simulink model "Case_7bus"  (R2023b)
settings: Solver=FixedStepAuto  StartTime=0  StopTime=4  FixedStep=Ts  RelTol=1e-3
PreLoadFcn:
  | FS_Frequency=csvread('FSConfig.csv',1,0); clear FS_Result FS_Freq_point; Noise_amp=0.5e-3;load("Dome/Case_7bus/XInitial7.mat");
InitFcn:
  | FS_Frequency=csvread('FSConfig.csv',1,0); clear FS_Result FS_Freq_point; Noise_amp=0.5e-3;load("Dome/Case_7bus/XInitial7.mat");
StartFcn:
  | FS_Frequency=csvread('FSConfig.csv',1,0); clear FS_Result FS_Freq_point; Noise_amp=0.5e-3;load("Dome/Case_7bus/XInitial7.mat");
undefined symbols (not defined in the file or in its folder): ApparatusDiscreDamping, ApparatusPara, ApparatusPowerFlow, ApparatusType, OtherInputs, Ts, Wbase, x_e, Ybase, Zbase
libraries: SimplusGT x20, spsGroundLib x13, spsThreePhaseParallelRLCBranchLib x7, spsThreePhaseSeriesRLCBranchLib x7, dspindex x4, spsControlledVoltageSourceLib x3, dspsnks4 x2, simulink x1, sps_lib x1
settings Model: Creator=yz34218  LastModifiedBy=yz34218
settings DataIOCC: InitialState=XInitial7  LoadInitialState=on

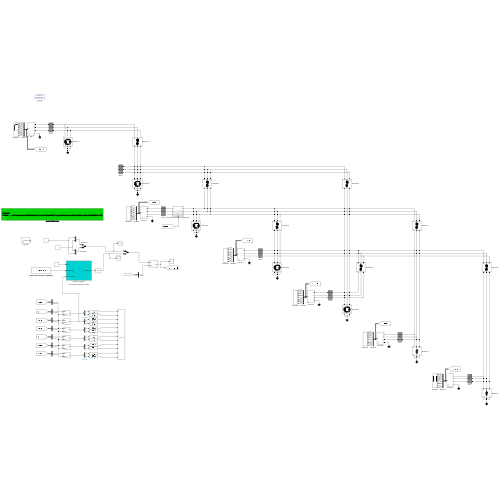
[thumbnail: Simulink's stored preview of the top-level diagram]
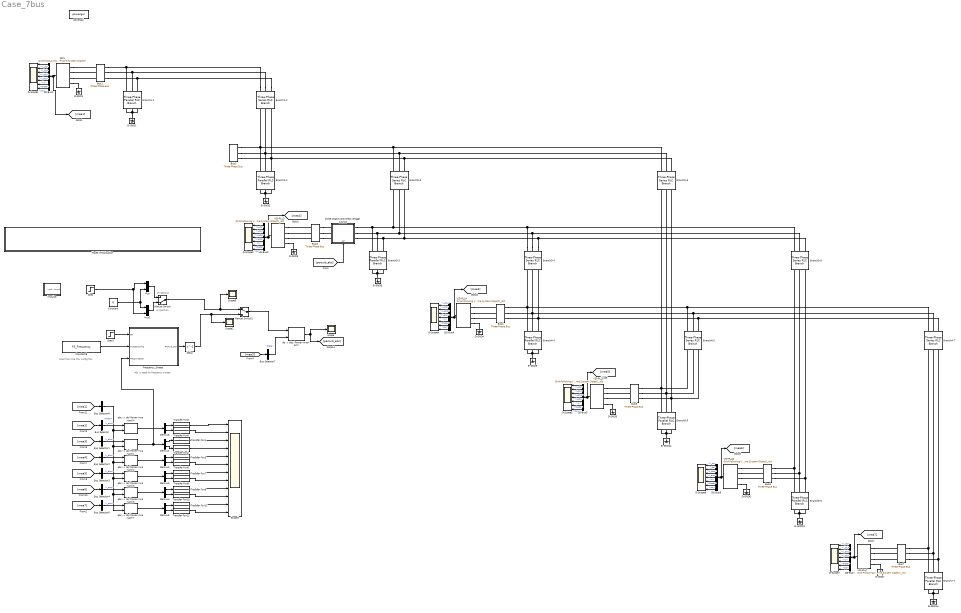
== system Case_7bus ==
  note: d-injection
  note: q-injection
  note: 40s is need for frequency sweep
  note: Input from the CSV config file.
  B-GND{1,3,6,9,12..14} (7 alike) : spsGroundLib/Ground  LConnTagsString=a
  Branch1-1 : spsThreePhaseParallelRLCBranchLib/Three-Phase Parallel RLC Branch  LConnTagsString=A|B|C  RConnTagsString=A|B|C  BranchType=RC  Resistance=(0.15273)*Zbase  Inductance=(Inf)*Zbase/Wbase  Capacitance=(0.042)*Ybase/Wbase  Measurements=None
  Branch1-2 : spsThreePhaseSeriesRLCBranchLib/Three-Phase Series RLC Branch  LConnTagsString=A|B|C  RConnTagsString=A|B|C  BranchType=RL  Resistance=(1e-06)*Zbase  Inductance=(0.039)*Zbase/Wbase  Capacitance=1e-6  Measurements=None
  Branch2-2 : spsThreePhaseParallelRLCBranchLib/Three-Phase Parallel RLC Branch  LConnTagsString=A|B|C  RConnTagsString=A|B|C  BranchType=RC  Resistance=(0.32435)*Zbase  Inductance=(Inf)*Zbase/Wbase  Capacitance=(0.042967)*Ybase/Wbase  Measurements=None
  Branch2-3 : spsThreePhaseSeriesRLCBranchLib/Three-Phase Series RLC Branch  LConnTagsString=A|B|C  RConnTagsString=A|B|C  BranchType=RL  Resistance=(0.015)*Zbase  Inductance=(0.225)*Zbase/Wbase  Capacitance=1e-6  Measurements=None
  Branch2-5 : spsThreePhaseSeriesRLCBranchLib/Three-Phase Series RLC Branch  LConnTagsString=A|B|C  RConnTagsString=A|B|C  BranchType=RL  Resistance=(0.0038)*Zbase  Inductance=(0.049)*Zbase/Wbase  Capacitance=1e-6  Measurements=None
  Branch3-3 : spsThreePhaseParallelRLCBranchLib/Three-Phase Parallel RLC Branch  LConnTagsString=A|B|C  RConnTagsString=A|B|C  BranchType=RC  Resistance=(1.4582)*Zbase  Inductance=(Inf)*Zbase/Wbase  Capacitance=(0.1491)*Ybase/Wbase  Measurements=None
  Branch3-4 : spsThreePhaseSeriesRLCBranchLib/Three-Phase Series RLC Branch  LConnTagsString=A|B|C  RConnTagsString=A|B|C  BranchType=RL  Resistance=(0.005)*Zbase  Inductance=(0.076)*Zbase/Wbase  Capacitance=1e-6  Measurements=None
  Branch3-6 : spsThreePhaseSeriesRLCBranchLib/Three-Phase Series RLC Branch  LConnTagsString=A|B|C  RConnTagsString=A|B|C  BranchType=RL  Resistance=(0.002)*Zbase  Inductance=(0.02)*Zbase/Wbase  Capacitance=1e-6  Measurements=None
  Branch4-4 : spsThreePhaseParallelRLCBranchLib/Three-Phase Parallel RLC Branch  LConnTagsString=A|B|C  RConnTagsString=A|B|C  BranchType=RC  Resistance=(1.4454)*Zbase  Inductance=(Inf)*Zbase/Wbase  Capacitance=(0.1142)*Ybase/Wbase  Measurements=None
  Branch4-5 : spsThreePhaseSeriesRLCBranchLib/Three-Phase Series RLC Branch  LConnTagsString=A|B|C  RConnTagsString=A|B|C  BranchType=RL  Resistance=(0.003)*Zbase  Inductance=(0.038)*Zbase/Wbase  Capacitance=1e-6  Measurements=None
  Branch4-7 : spsThreePhaseSeriesRLCBranchLib/Three-Phase Series RLC Branch  LConnTagsString=A|B|C  RConnTagsString=A|B|C  BranchType=RL  Resistance=(0.004)*Zbase  Inductance=(0.04)*Zbase/Wbase  Capacitance=1e-6  Measurements=None
  Branch5-5 : spsThreePhaseParallelRLCBranchLib/Three-Phase Parallel RLC Branch  LConnTagsString=A|B|C  RConnTagsString=A|B|C  BranchType=RC  Resistance=(2.3723)*Zbase  Inductance=(Inf)*Zbase/Wbase  Capacitance=(0.1792)*Ybase/Wbase  Measurements=None
  Branch6-6 : spsThreePhaseParallelRLCBranchLib/Three-Phase Parallel RLC Branch  LConnTagsString=A|B|C  RConnTagsString=A|B|C  BranchType=C  Resistance=(Inf)*Zbase  Inductance=(Inf)*Zbase/Wbase  Capacitance=(0.2)*Ybase/Wbase  Measurements=None
  Branch7-7 : spsThreePhaseParallelRLCBranchLib/Three-Phase Parallel RLC Branch  LConnTagsString=A|B|C  RConnTagsString=A|B|C  BranchType=C  Resistance=(Inf)*Zbase  Inductance=(Inf)*Zbase/Wbase  Capacitance=(0.2)*Ybase/Wbase  Measurements=None
  Bus Selector{,1..5} (6 alike) : BusSelector  OutputSignals=i_abc
  Bus Selector6 : BusSelector  OutputSignals=theta
  Bus Selector7 : BusSelector  OutputSignals=theta
  Bus{1..7} (7 alike) : SimplusGT/Three-Phase Bus  Vbase=1  Sbase=1
      settings: SourceProductName=Simplus Grid Tool
  Constant : Constant  Value=0
  Constant8 : Constant  Value=FS_Frequency
  D-GND{1,3..7} (6 alike) : spsGroundLib/Ground  LConnTagsString=a
  D-Scope{1,3..7} (6 alike) : Scope  NumInputPorts=7
  DS-Bus{1,3..7} (6 alike) : BusSelector  OutputSignals=v_dq,i_dq,v_abc,i_abc,w,theta,pq
  Delay : Delay  DelayLength=1
  Demux{1..5,8} (6 alike) : Demux  Outputs=2
  Frequency_Sweep : Subsystem  mask{Gain=0.01, Interval=0}
      mask prompts: Gain "Output Gain"; Interval "Injection Interval"
  Manual Switch : ManualSwitch  CurrentSetting=0
  Manual Switch1 : ManualSwitch
  Model Initialization : Subsystem  mask(Model Functions){InitFcnVar=FS_Frequency=csvread('FSConfig.csv',1,0); clear FS_Result FS_Freq_point; Noise_amp=0.5e-3;load("Dome/Case_7bus/XInitial7.mat");}
      mask prompts: InitFcnVar "InitFcn"
      mask init:
      | set_param(bdroot, 'PreLoadFcn', InitFcnVar);
      | set_param(bdroot, 'InitFcn', InitFcnVar);
      | set_param(bdroot, 'StartFcn', InitFcnVar);
      | PLF = get_param(bdroot, 'PreLoadFcn');
      | IF = get_param(bdroot, 'InitFcn');
      | SF = get_param(bdroot, 'StartFcn');
      | 
      | 
      | pos = get_param(gcb, 'Position');
      | width = pos(3) - pos(1); height = pos(4) - pos(2);
      mask Display:
      | text(5, height*0.5, [ ...
      | upper(bdroot) '\n' ...
      | '- InitFcn. . . . . '  get_param(bdroot, 'InitFcn')  ...
      | ], ...
      | 'horizontalAlignment', 'left', 'verticalAlignment', 'middle') ;
  Mux : Mux  Inputs=2
  Mux1 : Mux  Inputs=2
  SM1 : SimplusGT/Synchronous Machine (dq-Frame System Object)  Ts=Ts  Sbase=Sbase  Vbase=Vbase  Wbase=Wbase  ApparatusType=ApparatusType{1}  ApparatusPara=ApparatusPara{1}  PowerFlow=ApparatusPowerFlow{1}  x0=x_e{1}  OtherInputs=OtherInputs{1}  DiscreMethod=Hybrid Trapezoidal  EnableInsideModification=off  DiscreDampingFlag=on  DiscreDampingValue=ApparatusDiscreDamping{1}  LinearizationTimes=1  DirectFeedthrough=off
      settings: SourceProductName=Simplus Grid Tool
  Scope : Scope
  Scope2 : Scope
  Scope3 : Scope  NumInputPorts=12
  Scope5 : Scope
  Step : Step  After=2e-2  SampleTime=0
  Step1 : Step  Time=2  SampleTime=0
  Transfer Fcn{1..12} (12 alike) : TransferFcn  Denominator=[1/(2*pi*200) 1]
  VSI-PLL3 : SimplusGT/Grid-Following Voltage-Source Inverter (dq-Frame System Object)_old  Ts=Ts  Sbase=Sbase  Vbase=Vbase  Wbase=Wbase  ApparatusType=ApparatusType{3}  ApparatusPara=ApparatusPara{3}  PowerFlow=ApparatusPowerFlow{3}  x0=x_e{3}  OtherInputs=OtherInputs{3}  DiscreMethod=Hybrid Trapezoidal  EnableInsideModification=off  DiscreDampingFlag=on  DiscreDampingValue=ApparatusDiscreDamping{3}  LinearizationTimes=1  DirectFeedthrough=off
      settings: SourceProductName=Simplus Grid Tool
  VSI-PLL4 : SimplusGT/Grid-Following Voltage-Source Inverter (dq-Frame System Object)_old  Ts=Ts  Sbase=Sbase  Vbase=Vbase  Wbase=Wbase  ApparatusType=ApparatusType{4}  ApparatusPara=ApparatusPara{4}  PowerFlow=ApparatusPowerFlow{4}  x0=x_e{4}  OtherInputs=OtherInputs{4}  DiscreMethod=Hybrid Trapezoidal  EnableInsideModification=off  DiscreDampingFlag=on  DiscreDampingValue=ApparatusDiscreDamping{4}  LinearizationTimes=1  DirectFeedthrough=off
      settings: SourceProductName=Simplus Grid Tool
  VSI-PLL5 : SimplusGT/Grid-Following Voltage-Source Inverter (dq-Frame System Object)_old  Ts=Ts  Sbase=Sbase  Vbase=Vbase  Wbase=Wbase  ApparatusType=ApparatusType{5}  ApparatusPara=ApparatusPara{5}  PowerFlow=ApparatusPowerFlow{5}  x0=x_e{5}  OtherInputs=OtherInputs{5}  DiscreMethod=Hybrid Trapezoidal  EnableInsideModification=off  DiscreDampingFlag=on  DiscreDampingValue=ApparatusDiscreDamping{5}  LinearizationTimes=1  DirectFeedthrough=off
      settings: SourceProductName=Simplus Grid Tool
  VSI-PLL6 : SimplusGT/Grid-Following Voltage-Source Inverter (dq-Frame System Object)_old  Ts=Ts  Sbase=Sbase  Vbase=Vbase  Wbase=Wbase  ApparatusType=ApparatusType{6}  ApparatusPara=ApparatusPara{6}  PowerFlow=ApparatusPowerFlow{6}  x0=x_e{6}  OtherInputs=OtherInputs{6}  DiscreMethod=Hybrid Trapezoidal  EnableInsideModification=off  DiscreDampingFlag=on  DiscreDampingValue=ApparatusDiscreDamping{6}  LinearizationTimes=1  DirectFeedthrough=off
      settings: SourceProductName=Simplus Grid Tool
  VSI-PLL7 : SimplusGT/Grid-Following Voltage-Source Inverter (dq-Frame System Object)_old  Ts=Ts  Sbase=Sbase  Vbase=Vbase  Wbase=Wbase  ApparatusType=ApparatusType{7}  ApparatusPara=ApparatusPara{7}  PowerFlow=ApparatusPowerFlow{7}  x0=x_e{7}  OtherInputs=OtherInputs{7}  DiscreMethod=Hybrid Trapezoidal  EnableInsideModification=off  DiscreDampingFlag=on  DiscreDampingValue=ApparatusDiscreDamping{7}  LinearizationTimes=1  DirectFeedthrough=off
      settings: SourceProductName=Simplus Grid Tool
  abc -> dq (Power-Invariant){1..4,6..7} (6 alike) : SimplusGT/abc -> dq (Power-Invariant)  SystemSampleTime=-1  VariantActivationTime=update diagram  AllowFlexibleInterface=on  Latency=0  AutoFrameSizeCalculation=off
      settings: SourceProductName=Simplus Grid Tool
  "dq -> abc (Power-Invariant)" : SimplusGT/dq -> abc (Power-Invariant)  SystemSampleTime=-1  VariantActivationTime=update diagram  AllowFlexibleInterface=on  Latency=0  AutoFrameSizeCalculation=off
      settings: SourceProductName=Simplus Grid Tool
  impulse : Subsystem  mask{Amp=2e-2, Tstart=1, Ti=1e-3}
      mask prompts: Amp "amplitude"; Ti "Tinterval"
  powergui : sps_lib/powergui  Priority=1  SimulationMode=Discrete  SampleTime=Ts  frequency=60  Iterations=50  frequencyindice=0  Pbase=100e6  ErrMax=1e-4  UnitsV=kV  UnitsW=MW  buscounter=0  FunctionMessages=off  echomessages=off  EnableUseOfTLC=off  CurrentSourceSwitches=off  DisableSnubberDevices=off  DisableRonSwitches=off  DisableVfSwitches=off  DisplayEquations=off  AutomaticDiscreteSolvers=off  SolverType=Tustin/Backward Euler (TBE)  Interpol=off  ExternalGateDelay=off  methode=off  Ts=100  x0status=blocks  SPID=on  SwTol=0  HookPort=off  NonlinearTolerance=1e-4  nMaxIteration=100  ContinueOnMaxIteration=off  RestoreLinks=warning  ResistiveCurrentMeasurement=off  Frange=[0:2:500]  Ylog=off  Xlog=on  ShowGrid=off  save=off  variable=ZData  structure=0  ZoomFFT=off  StartTime=0.0  cycles=1  DisplayStyle=1  fundamental=60  FreqAxis=off  MaxFrequency=1000  frequencyindicesteady=1  RmsSteady=1  display=off
  three-phase controlled voltage source : Subsystem
      settings: PortSchema="{\"entries\":[{\"content\":{\"sides\":[{\"content\":{\"connectorIds\":[\"LConn1\",\"LConn2\",\"LConn3\"]},\"type\":\"ConnectorPlacement.EquallySpacedRectSide\",\"uuid\":\"6f603e87-6b2e-4585-ad3a-55936445c397\"},{\"content\":{\"connectorIds\":[\"RConn1\",\"RConn2\",\"RConn3\"],\"side\":\"RIGHT\"},\"type\":\"ConnectorPlacement.EquallySpacedRectSide\",\"uuid\":\"08c5aebc-ed45-455a-9198-e657d358a757\"},{\"content\":{\"side\":\"TOP\"},\"type\":\"ConnectorPlacement.EquallySpacedRectSide\",\"uuid\":\"90e892ab-d7d1-4f2e-b125-0b742fd1657c\"},{\"content\":{\"connectorIds\":[\"In1\"],\"side\":\"BOTTOM\"},\"type\":\"ConnectorPlacement.EquallySpacedRectSide\",\"uuid\":\"ba12d237-2ee0-4e5a-b3d4-1de3f90cbef1\"}]},\"type\":\"ConnectorPlacement.EquallySpacedConnector\",\"uuid\":\"0150c08c-ed05-4e99-aa85-f9e708dbbe93\"}],\"packageUris\":[\"http://schema.mathworks.com/mf0/Connector/R2020b\"],\"version\":\"1.0\"}"
  wires:
  SM1/1 -> [mea1], DS-Bus1/1
  DS-Bus1/1 -> D-Scope1/1  "<v_dq>"
  DS-Bus1/2 -> D-Scope1/2  "<i_dq>"
  DS-Bus1/3 -> D-Scope1/3  "<v_abc>"
  DS-Bus1/4 -> D-Scope1/4  "<i_abc>"
  DS-Bus1/5 -> D-Scope1/5  "<w>"
  DS-Bus1/6 -> D-Scope1/6  "<theta>"
  DS-Bus1/7 -> D-Scope1/7  "<pq>"
  VSI-PLL3/1 -> [mea3], DS-Bus3/1
  DS-Bus3/1 -> D-Scope3/1  "<v_dq>"
  DS-Bus3/2 -> D-Scope3/2  "<i_dq>"
  DS-Bus3/3 -> D-Scope3/3  "<v_abc>"
  DS-Bus3/4 -> D-Scope3/4  "<i_abc>"
  DS-Bus3/5 -> D-Scope3/5  "<w>"
  DS-Bus3/6 -> D-Scope3/6  "<theta>"
  DS-Bus3/7 -> D-Scope3/7  "<pq>"
  VSI-PLL4/1 -> [mea4], DS-Bus4/1
  DS-Bus4/1 -> D-Scope4/1  "<v_dq>"
  DS-Bus4/2 -> D-Scope4/2  "<i_dq>"
  DS-Bus4/3 -> D-Scope4/3  "<v_abc>"
  DS-Bus4/4 -> D-Scope4/4  "<i_abc>"
  DS-Bus4/5 -> D-Scope4/5  "<w>"
  DS-Bus4/6 -> D-Scope4/6  "<theta>"
  DS-Bus4/7 -> D-Scope4/7  "<pq>"
  VSI-PLL5/1 -> [mea5], DS-Bus5/1
  DS-Bus5/1 -> D-Scope5/1  "<v_dq>"
  DS-Bus5/2 -> D-Scope5/2  "<i_dq>"
  DS-Bus5/3 -> D-Scope5/3  "<v_abc>"
  DS-Bus5/4 -> D-Scope5/4  "<i_abc>"
  DS-Bus5/5 -> D-Scope5/5  "<w>"
  DS-Bus5/6 -> D-Scope5/6  "<theta>"
  DS-Bus5/7 -> D-Scope5/7  "<pq>"
  VSI-PLL6/1 -> [mea6], DS-Bus6/1
  DS-Bus6/1 -> D-Scope6/1  "<v_dq>"
  DS-Bus6/2 -> D-Scope6/2  "<i_dq>"
  DS-Bus6/3 -> D-Scope6/3  "<v_abc>"
  DS-Bus6/4 -> D-Scope6/4  "<i_abc>"
  DS-Bus6/5 -> D-Scope6/5  "<w>"
  DS-Bus6/6 -> D-Scope6/6  "<theta>"
  DS-Bus6/7 -> D-Scope6/7  "<pq>"
  VSI-PLL7/1 -> [mea7], DS-Bus7/1
  DS-Bus7/1 -> D-Scope7/1  "<v_dq>"
  DS-Bus7/2 -> D-Scope7/2  "<i_dq>"
  DS-Bus7/3 -> D-Scope7/3  "<v_abc>"
  DS-Bus7/4 -> D-Scope7/4  "<i_abc>"
  DS-Bus7/5 -> D-Scope7/5  "<w>"
  DS-Bus7/6 -> D-Scope7/6  "<theta>"
  DS-Bus7/7 -> D-Scope7/7  "<pq>"
  [perturb_abc] -> three-phase controlled voltage source/1(ref)
  Frequency_Sweep/1(Perturb_DQ) -> Delay/1
  Manual Switch/1 -> Scope5/1, Manual Switch1/1
  Constant8/1 -> Frequency_Sweep/2(SweepConfig)
  Mux/1 -> Manual Switch/1
  Step/1 -> Mux1/2, Mux/1
  Delay/1 -> Scope2/1, Manual Switch1/2
  Step1/1 -> Frequency_Sweep/1(EN)
  Manual Switch1/1 -> "dq -> abc (Power-Invariant)"/1
  "dq -> abc (Power-Invariant)"/1 -> Scope/1, [perturb_abc]
  Constant/1 -> Mux/2, Mux1/1
  "abc -> dq (Power-Invariant)1"/1 -> Frequency_Sweep/3(ResponseDQ), Demux1/1
  Mux1/1 -> Manual Switch/2
  [mea1] -> Bus Selector/1
  [mea3] -> Bus Selector1/1
  [mea4] -> Bus Selector2/1
  [mea5] -> Bus Selector3/1
  [mea6] -> Bus Selector4/1
  [mea7] -> Bus Selector5/1
  [mea1] -> Bus Selector6/1
  Bus Selector/1 -> "abc -> dq (Power-Invariant)4"/1  "<i_abc>"
  Bus Selector1/1 -> "abc -> dq (Power-Invariant)1"/1  "<i_abc>"
  Bus Selector2/1 -> "abc -> dq (Power-Invariant)2"/1  "<i_abc>"
  Bus Selector3/1 -> "abc -> dq (Power-Invariant)3"/1  "<i_abc>"
  Bus Selector4/1 -> "abc -> dq (Power-Invariant)6"/1  "<i_abc>"
  Bus Selector5/1 -> "abc -> dq (Power-Invariant)7"/1  "<i_abc>"
  Bus Selector6/1 -> "abc -> dq (Power-Invariant)7"/2, "abc -> dq (Power-Invariant)6"/2, "abc -> dq (Power-Invariant)3"/2, "abc -> dq (Power-Invariant)2"/2, "abc -> dq (Power-Invariant)1"/2, "abc -> dq (Power-Invariant)4"/2  "<theta>"
  "abc -> dq (Power-Invariant)4"/1 -> Demux8/1
  "abc -> dq (Power-Invariant)2"/1 -> Demux2/1
  "abc -> dq (Power-Invariant)3"/1 -> Demux3/1
  "abc -> dq (Power-Invariant)6"/1 -> Demux4/1
  "abc -> dq (Power-Invariant)7"/1 -> Demux5/1
  Demux8/1 -> Transfer Fcn3/1
  Demux8/2 -> Transfer Fcn4/1
  Demux2/1 -> Transfer Fcn5/1
  Demux2/2 -> Transfer Fcn6/1
  Demux3/1 -> Transfer Fcn7/1
  Demux3/2 -> Transfer Fcn8/1
  Demux4/1 -> Transfer Fcn9/1
  Demux4/2 -> Transfer Fcn10/1
  Demux5/1 -> Transfer Fcn11/1
  Demux5/2 -> Transfer Fcn12/1
  [mea3] -> Bus Selector7/1
  Bus Selector7/1 -> "dq -> abc (Power-Invariant)"/2  "<theta>"
  Demux1/1 -> Transfer Fcn1/1
  Transfer Fcn1/1 -> Scope3/3
  Demux1/2 -> Transfer Fcn2/1
  Transfer Fcn2/1 -> Scope3/4
  Transfer Fcn3/1 -> Scope3/1
  Transfer Fcn4/1 -> Scope3/2
  Transfer Fcn5/1 -> Scope3/5
  Transfer Fcn6/1 -> Scope3/6
  Transfer Fcn7/1 -> Scope3/7
  Transfer Fcn8/1 -> Scope3/8
  Transfer Fcn9/1 -> Scope3/9
  Transfer Fcn10/1 -> Scope3/10
  Transfer Fcn11/1 -> Scope3/11
  Transfer Fcn12/1 -> Scope3/12
  connections:
  SM1/LConn4 -- D-GND1/LConn1
  VSI-PLL3/LConn4 -- D-GND3/LConn1
  VSI-PLL4/LConn4 -- D-GND4/LConn1
  VSI-PLL5/LConn4 -- D-GND5/LConn1
  VSI-PLL6/LConn4 -- D-GND6/LConn1
  VSI-PLL7/LConn4 -- D-GND7/LConn1
  Branch1-1/RConn1 -- Branch1-1/RConn2 -- Branch1-1/RConn3 -- B-GND1/LConn1
  Branch2-2/RConn1 -- Branch2-2/RConn2 -- Branch2-2/RConn3 -- B-GND3/LConn1
  Branch3-3/RConn1 -- Branch3-3/RConn2 -- Branch3-3/RConn3 -- B-GND6/LConn1
  Branch4-4/RConn1 -- Branch4-4/RConn2 -- Branch4-4/RConn3 -- B-GND9/LConn1
  Branch5-5/RConn1 -- Branch5-5/RConn2 -- Branch5-5/RConn3 -- B-GND12/LConn1
  Branch6-6/RConn1 -- Branch6-6/RConn2 -- Branch6-6/RConn3 -- B-GND13/LConn1
  Branch7-7/RConn1 -- Branch7-7/RConn2 -- Branch7-7/RConn3 -- B-GND14/LConn1
  Branch1-2/RConn1 -- Bus2/RConn1 -- Branch2-2/LConn1 -- Branch2-5/LConn1 -- Branch2-3/LConn1
  Branch1-2/RConn2 -- Bus2/RConn2 -- Branch2-2/LConn2 -- Branch2-5/LConn2 -- Branch2-3/LConn2
  Branch1-2/RConn3 -- Bus2/RConn3 -- Branch2-2/LConn3 -- Branch2-5/LConn3 -- Branch2-3/LConn3
  Branch1-2/LConn1 -- Bus1/RConn1 -- Branch1-1/LConn1
  Branch1-2/LConn2 -- Bus1/RConn2 -- Branch1-1/LConn2
  Branch1-2/LConn3 -- Bus1/RConn3 -- Branch1-1/LConn3
  Branch3-4/LConn1 -- three-phase controlled voltage source/RConn1 -- Branch3-3/LConn1 -- Branch2-3/RConn1 -- Branch3-6/LConn1
  Branch3-4/LConn2 -- three-phase controlled voltage source/RConn2 -- Branch3-3/LConn2 -- Branch2-3/RConn2 -- Branch3-6/LConn2
  Branch3-4/LConn3 -- three-phase controlled voltage source/RConn3 -- Branch3-3/LConn3 -- Branch2-3/RConn3 -- Branch3-6/LConn3
  Branch2-5/RConn1 -- Bus5/RConn1 -- Branch5-5/LConn1 -- Branch4-5/RConn1
  Branch2-5/RConn2 -- Bus5/RConn2 -- Branch5-5/LConn2 -- Branch4-5/RConn2
  Branch2-5/RConn3 -- Bus5/RConn3 -- Branch5-5/LConn3 -- Branch4-5/RConn3
  Branch3-4/RConn1 -- Bus4/RConn1 -- Branch4-4/LConn1 -- Branch4-7/LConn1 -- Branch4-5/LConn1
  Branch3-4/RConn2 -- Bus4/RConn2 -- Branch4-4/LConn2 -- Branch4-7/LConn2 -- Branch4-5/LConn2
  Branch3-4/RConn3 -- Bus4/RConn3 -- Branch4-4/LConn3 -- Branch4-7/LConn3 -- Branch4-5/LConn3
  Branch3-6/RConn1 -- Bus6/RConn1 -- Branch6-6/LConn1
  Branch3-6/RConn2 -- Bus6/RConn2 -- Branch6-6/LConn2
  Branch3-6/RConn3 -- Bus6/RConn3 -- Branch6-6/LConn3
  Branch4-7/RConn1 -- Bus7/RConn1 -- Branch7-7/LConn1
  Branch4-7/RConn2 -- Bus7/RConn2 -- Branch7-7/LConn2
  Branch4-7/RConn3 -- Bus7/RConn3 -- Branch7-7/LConn3
  SM1/LConn1 -- Bus1/LConn1
  SM1/LConn2 -- Bus1/LConn2
  SM1/LConn3 -- Bus1/LConn3
  VSI-PLL3/LConn1 -- Bus3/LConn1
  VSI-PLL3/LConn2 -- Bus3/LConn2
  VSI-PLL3/LConn3 -- Bus3/LConn3
  VSI-PLL4/LConn1 -- Bus4/LConn1
  VSI-PLL4/LConn2 -- Bus4/LConn2
  VSI-PLL4/LConn3 -- Bus4/LConn3
  VSI-PLL5/LConn1 -- Bus5/LConn1
  VSI-PLL5/LConn2 -- Bus5/LConn2
  VSI-PLL5/LConn3 -- Bus5/LConn3
  VSI-PLL6/LConn1 -- Bus6/LConn1
  VSI-PLL6/LConn2 -- Bus6/LConn2
  VSI-PLL6/LConn3 -- Bus6/LConn3
  VSI-PLL7/LConn1 -- Bus7/LConn1
  VSI-PLL7/LConn2 -- Bus7/LConn2
  VSI-PLL7/LConn3 -- Bus7/LConn3
  Bus3/RConn1 -- three-phase controlled voltage source/LConn1
  Bus3/RConn2 -- three-phase controlled voltage source/LConn2
  Bus3/RConn3 -- three-phase controlled voltage source/LConn3

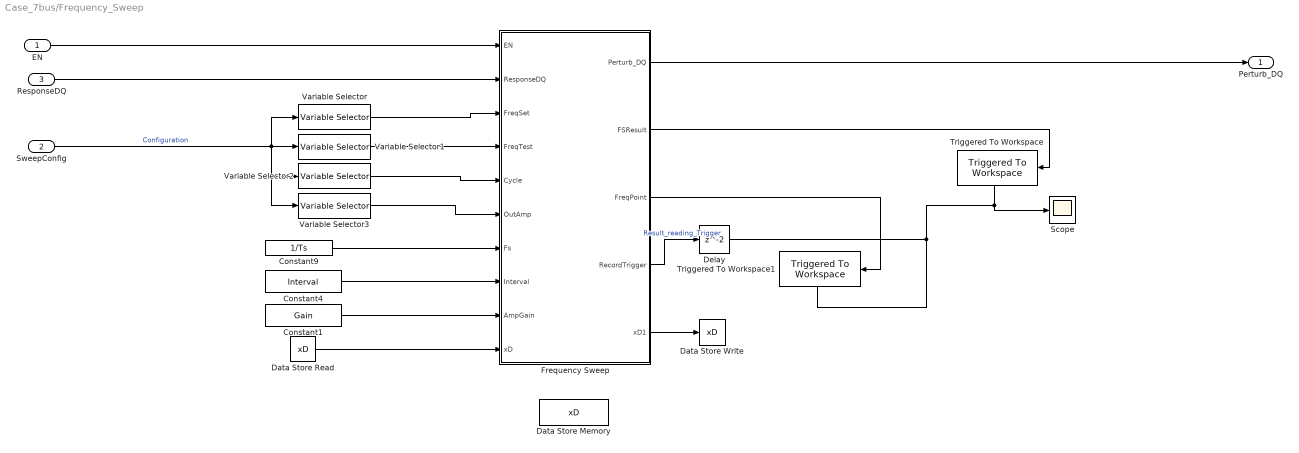
== system Case_7bus/Frequency_Sweep ==
  EN : Inport
  SweepConfig : Inport  Port=2
  ResponseDQ : Inport  Port=3
  Constant1 : Constant  Value=Gain
  Constant4 : Constant  Value=Interval
  Constant9 : Constant  Value=1/Ts
  Data Store Memory : DataStoreMemory  DataStoreName=xD  WriteAfterWriteMsg=warning  InitialValue=zeros(1,16)  ShowAdditionalParam=off
  Data Store Read : DataStoreRead  DataStoreName=xD  IndexOptions=Index vector (dialog)  Indices=1  OutputSizes=1
  Data Store Write : DataStoreWrite  DataStoreName=xD  IndexOptions=Index vector (dialog)  Indices=1  OutputSizes=1
  Delay : Delay
  Frequency Sweep : MATLAB Function  TreatAsAtomicUnit=on
  Scope : Scope
  Triggered To Workspace : dspsnks4/Triggered To Workspace  TriggerType=Rising edge  VariableName=FS_Result  Buffer=5000  Save2DMode=2-D array (concatenate along first dimension)
      settings: FixptAsFi=off
  Triggered To Workspace1 : dspsnks4/Triggered To Workspace  TriggerType=Rising edge  VariableName=FS_Freq_point  Buffer=5000  Save2DMode=2-D array (concatenate along first dimension)
      settings: FixptAsFi=off
  Variable Selector : dspindex/Variable Selector  NumInputs=1  rowsOrCols=Columns  IdxMode=Fixed  Elements=1  ZerOneIdxMode=One-based  errmode=Clip Index  FillMode=on  FillValues=0
  Variable Selector1 : dspindex/Variable Selector  NumInputs=1  rowsOrCols=Columns  IdxMode=Fixed  Elements=2  ZerOneIdxMode=One-based  errmode=Clip Index  FillMode=on  FillValues=0
  Variable Selector2 : dspindex/Variable Selector  NumInputs=1  rowsOrCols=Columns  IdxMode=Fixed  Elements=3  ZerOneIdxMode=One-based  errmode=Clip Index  FillMode=on  FillValues=0
  Variable Selector3 : dspindex/Variable Selector  NumInputs=1  rowsOrCols=Columns  IdxMode=Fixed  Elements=4  ZerOneIdxMode=One-based  errmode=Clip Index  FillMode=on  FillValues=0
  Perturb_DQ : Outport
  wires:
  Variable Selector2/1 -> Frequency Sweep/5(Cycle)
  Frequency Sweep/2(FSResult) -> Triggered To Workspace/1
  Frequency Sweep/4(RecordTrigger) -> Delay/1  "Result_reading_Trigger"
  Constant4/1 -> Frequency Sweep/8(Interval)
  Frequency Sweep/5(xD1) -> Data Store Write/1
  Variable Selector3/1 -> Frequency Sweep/6(OutAmp)
  Variable Selector1/1 -> Frequency Sweep/4(FreqTest)
  SweepConfig/1 -> Variable Selector3/1, Variable Selector2/1, Variable Selector1/1, Variable Selector/1  "Configuration"
  ResponseDQ/1 -> Frequency Sweep/2(ResponseDQ)
  Variable Selector/1 -> Frequency Sweep/3(FreqSet)
  Frequency Sweep/3(FreqPoint) -> Triggered To Workspace1/1
  Data Store Read/1 -> Frequency Sweep/10(xD)
  Constant9/1 -> Frequency Sweep/7(Fs)
  Frequency Sweep/1(Perturb_DQ) -> Perturb_DQ/1
  EN/1 -> Frequency Sweep/1(EN)
  Delay/1 -> Triggered To Workspace/Trigger, Scope/1, Triggered To Workspace1/Trigger
  Constant1/1 -> Frequency Sweep/9(AmpGain)

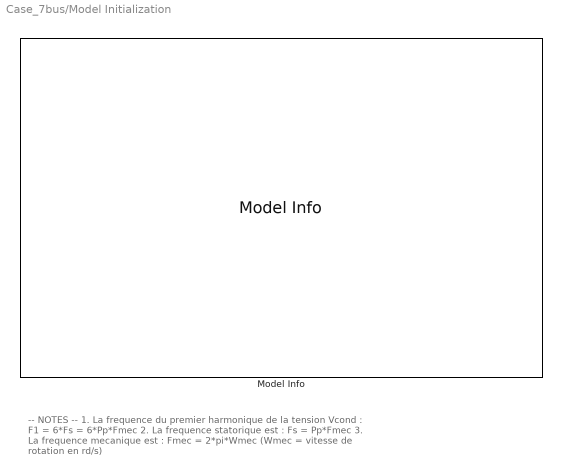
== system Case_7bus/Model Initialization ==
  note: -- NOTES --
      | 1. La frequence du premier harmonique de la tension Vcond :
      |     F1 = 6*Fs = 6*Pp*Fmec
      | 2. La frequence statorique est :
      |     Fs = Pp*Fmec
      | 3. La frequence mecanique est :
      |     Fmec = 2*pi*Wmec  (Wmec = vitesse de rotation en rd/s)
  Model Info : simulink/Model-Wide Utilities/Model Info  Frame=on  DisplayStringWithTags=|  HorizontalTextAlignment=Left  LeftAlignmentValue=0.02
      | - Version <<< %<ModelVersion> >>>
      | 
      | - Description :
      | %<Description>
      | 
      | - Created by :     %<Creator>
      | - Creation date : %<Created>
      | - Modified by :    %<ModifiedBy>
      | - Last modif. :     %<LastModificationDate>

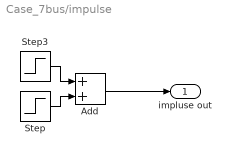
== system Case_7bus/impulse ==
  Add : Sum
  Step : Step  Time=Tstart+Ti  After=-Amp  SampleTime=0
  Step3 : Step  Time=Tstart  After=Amp  SampleTime=0
  impluse out : Outport
  wires:
  Step/1 -> Add/2
  Step3/1 -> Add/1
  Add/1 -> impluse out/1

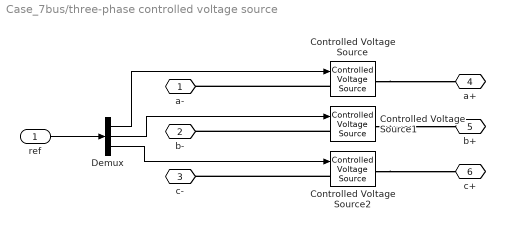
== system Case_7bus/three-phase controlled voltage source ==
  ref : Inport
  Controlled Voltage Source : spsControlledVoltageSourceLib/Controlled Voltage Source  Initialize=on  Source_Type=AC  Amplitude=0  Phase=0  Frequency=0  Measurements=None
  Controlled Voltage Source1 : spsControlledVoltageSourceLib/Controlled Voltage Source  Initialize=on  Source_Type=AC  Amplitude=0  Phase=0  Frequency=0  Measurements=None
  Controlled Voltage Source2 : spsControlledVoltageSourceLib/Controlled Voltage Source  Initialize=on  Source_Type=AC  Amplitude=0  Phase=0  Frequency=0  Measurements=None
  Demux : Demux  Outputs=3
  a- : PMIOPort  Side=Left
  b- : PMIOPort  Port=2  Side=Left
  c- : PMIOPort  Port=3  Side=Left
  a+ : PMIOPort  Port=4  Side=Right
  b+ : PMIOPort  Port=5  Side=Right
  c+ : PMIOPort  Port=6  Side=Right
  wires:
  Demux/2 -> Controlled Voltage Source1/1
  Demux/3 -> Controlled Voltage Source2/1
  ref/1 -> Demux/1
  Demux/1 -> Controlled Voltage Source/1
  connections:
  Controlled Voltage Source/LConn1 -- a-/RConn1
  Controlled Voltage Source1/RConn1 -- b+/RConn1
  Controlled Voltage Source1/LConn1 -- b-/RConn1
  Controlled Voltage Source/RConn1 -- a+/RConn1
  Controlled Voltage Source2/RConn1 -- c+/RConn1
  Controlled Voltage Source2/LConn1 -- c-/RConn1

== matlab function Case_7bus/Frequency_Sweep/Frequency Sweep ==
  data: EN input; Perturb_DQ output; ResponseDQ input size=[1 2]; FreqSet input; FreqTest input; Cycle input; OutAmp input; Fs input; Interval input; AmpGain input; xD input; FSResult output; FreqPoint output; RecordTrigger output; xD1 output
function [Perturb_DQ, FSResult, FreqPoint, RecordTrigger, xD1] = fcn(EN,ResponseDQ, FreqSet, FreqTest, Cycle, OutAmp, Fs, Interval, AmpGain, xD)
% State variables:
% xD0: case;        xD1:N; total sample points for one period
% xD2:-N;           xD3:n ,sample point count      xD4:k, for cycle count
% xD5: Out_Re       xD6:Out_Im;
% xD7: Sum_Re_d      xD8:Sum_Im_d     xD9:Sum_Re_q     xD10:Sum_Im_q
% xD11, xD12, xD13, xD14----xD7,xD8,xD9,xD10 * dt
% xD15: t, for waiting

% read states
CaseK=xD(1); % case
Ns=xD(2); % total time steps for the set frequency
Nt=xD(3); % total time steps for the tested (calculated) frequency
n=xD(4); % sample point count
kc=xD(5);   % CycleCount
OutD=xD(6); %   Output
OutQ=xD(7);
SumDRe=xD(8); % Integration
SumDIm=xD(9);
SumQRe=xD(10);
SumQIm=xD(11);
FinalDRe=xD(12); % Final Result (complex number)
FinalDIm=xD(13);
FinalQRe=xD(14);
FinalQIm=xD(15);
TWait=xD(16); % wait time

FrequencyNum=length(FreqSet);

if AmpGain==0
    error('gain must not be zero');
end

%% Main Loop
if EN==0   % if Enable 0, reset all variables
    OutD=0;
    OutQ=0;
else
    switch CaseK
        case 0 % the very first round
            kc=1;
            CaseK=1;
        case 1
            if kc>FrequencyNum         %sweep finished. Go to case 9
                OutD=0;
                OutQ=0;   
                CaseK=9; 
            elseif Cycle(kc)==0  % if this frequency is skipped
                kc=kc+1;
            else   
                % prepare to sweep D axis this frequency
                SumDRe=0;
                SumDIm=0;
                SumQRe=0;
                SumQIm=0;
                TWait=0;
                n=0;
                % total time steps for this frequency
                Ns = Fs/FreqSet(kc)*Cycle(kc); % for output count
                Nt = Fs/FreqTest(kc)*Cycle(kc); % for frequency test count
                OutD=OutAmp(kc)*sin(2*pi*Cycle(kc)*n/Ns)*AmpGain;
                OutQ=0;
                n=n+1;
                CaseK=2;
            end
        case 2 % sweep D axis
            OutD=OutAmp(kc)*sin(2*pi*Cycle(kc)*n/Ns)*AmpGain;
        	OutQ=0;
            % D sum
            SumDRe = SumDRe + ResponseDQ(1) * sin(2*pi*Cycle(kc)*(n-1)/Nt);  % Nt is used here, means it is using the tested frequency specified.
            SumDIm = SumDIm + (-1)*ResponseDQ(1) * (-1)*cos(2*pi*Cycle(kc)*(n-1)/Nt);
            % Q sum
            SumQRe = SumQRe + ResponseDQ(2) * sin(2*pi*Cycle(kc)*(n-1)/Nt);
            SumQIm = SumQIm + (-1)*ResponseDQ(2) * (-1)*cos(2*pi*Cycle(kc)*(n-1)/Nt);
            
            if(n<Nt)
                n=n+1;
            else
                OutD=0;
                OutQ=0;
                CaseK=3;
            end
        case 3
            % Set Sweep Results
            FinalDRe = 2*SumDRe*FreqSet(kc)/Cycle(kc)/Fs/OutAmp(kc)/AmpGain;                      
            FinalDIm = 2*SumDIm*FreqSet(kc)/Cycle(kc)/Fs/OutAmp(kc)/AmpGain; 
            FinalQRe = 2*SumQRe*FreqSet(kc)/Cycle(kc)/Fs/OutAmp(kc)/AmpGain;  
            FinalQIm = 2*SumQIm*FreqSet(kc)/Cycle(kc)/Fs/OutAmp(kc)/AmpGain;
            if TWait<Fs*Interval
                TWait=TWait+1;
            else
                TWait=0;
                CaseK=4;
            end
        case 4
            SumDRe=0;
            SumDIm=0;
            SumQRe=0;
            SumQIm=0;
            TWait=0;
            n=0;
            % total time steps for this frequency
            Ns = Fs/FreqSet(kc)*Cycle(kc); % for output count
            Nt = Fs/FreqTest(kc)*Cycle(kc); % for frequency test count
            OutD=0;
            OutQ=OutAmp(kc)*sin(2*pi*Cycle(kc)*n/Ns)*AmpGain;
            n=n+1;
            CaseK=5;
        case 5
            OutD=0;
        	OutQ=OutAmp(kc)*sin(2*pi*Cycle(kc)*n/Ns)*AmpGain;
            % D sum
            SumDRe = SumDRe + ResponseDQ(1) * sin(2*pi*Cycle(kc)*(n-1)/Nt);  % Nt is used here, means it is using the tested frequency specified.
            SumDIm = SumDIm + (-1)*ResponseDQ(1) * (-1)*cos(2*pi*Cycle(kc)*(n-1)/Nt);
            % Q sum
            SumQRe = SumQRe + ResponseDQ(2) * sin(2*pi*Cycle(kc)*(n-1)/Nt);
            SumQIm = SumQIm + (-1)*ResponseDQ(2) * (-1)*cos(2*pi*Cycle(kc)*(n-1)/Nt);
            
            if(n<Nt)
                n=n+1;
            else
                OutD=0;
                OutQ=0;
                CaseK=6;
            end
        case 6
            % Set Sweep Results
            FinalDRe = 2*SumDRe*FreqSet(kc)/Cycle(kc)/Fs/OutAmp(kc)/AmpGain;                      
            FinalDIm = 2*SumDIm*FreqSet(kc)/Cycle(kc)/Fs/OutAmp(kc)/AmpGain; 
            FinalQRe = 2*SumQRe*FreqSet(kc)/Cycle(kc)/Fs/OutAmp(kc)/AmpGain;  
            FinalQIm = 2*SumQIm*FreqSet(kc)/Cycle(kc)/Fs/OutAmp(kc)/AmpGain;
            if TWait<Fs*Interval
                TWait=TWait+1;
            else
                TWait=0;
                kc=kc+1;
                CaseK=1;
            end
        case 9 % nothing
    end
end


%% set outputs
xD1=[CaseK,Ns,Nt,n,kc,OutD,OutQ,SumDRe,SumDIm,SumQRe,SumQIm,FinalDRe,FinalDIm,FinalQRe,FinalQIm,TWait]; % write states
Perturb_DQ=[OutD,OutQ];
1i;
if kc>0 && EN==1
    FSResult = [FinalDRe+FinalDIm*1i, FinalQRe+FinalQIm*1i]; % complex number output
    if kc>FrequencyNum
        kc=FrequencyNum;
    end
    FreqPoint = FreqSet(kc);
    % if TWait>=Fs*Interval/4 && TWait<Fs*Interval*3/4
    %     RecordTrigger=1;
    % else
    %     RecordTrigger=0;
    % end
else
    FSResult=[0,0];
    %RecordTrigger=0;
    FreqPoint=0;
end
if CaseK==3 || CaseK==6
    RecordTrigger=1; % trigger is deleyed for two cycles outside the block.
else
    RecordTrigger=0;
end

end
